simulink model "Standalone_CCSMPC_Controller"  (R2025b)
settings: Solver=FixedStepDiscrete  StartTime=0.0  StopTime=20  FixedStep=1e-4  MaxStep=1e-4  RelTol=1e-3
undefined symbols (not defined in the file): B_fric, J, Ld, Lq, PsiPM, Rs, Ts_ctrl, Ts_sim
libraries: simulink x1
settings Model: SimulationMode=processor-in-the-loop (pil)  Creator=Harish  LastModifiedBy=Harish
settings OptimizationCC: DefaultParameterBehavior=Inlined  EnhancedBackFolding=on  PassReuseOutputArgsAs=Individual arguments  ZeroExternalMemoryAtStartup=off  ZeroInternalMemoryAtStartup=off  OptimizeBlockOrder=speed  DifferentSizesBufferReuse=on  OptimizationCustomize=off  EfficientTunableParamExpr=on
settings DebuggingCC: ParameterTunabilityLossMsg=error
settings HardwareCC: TargetLargestAtomicInteger=Long  TargetLargestAtomicFloat=Double  TargetIntDivRoundTo=Zero  TargetEndianess=LittleEndian  TargetHWDeviceType=ARM Compatible->ARM Cortex-M
settings SFSimCC: MATLABDynamicMemAlloc=off
settings RTWCC: SystemTargetFile=ert.tlc  TemplateMakefile=ert_default_tmf  GenerateReport=on  Toolchain=MinGW64 | gmake (64-bit Windows)  GenerateCodeMetricsReport=on  Description=Embedded Coder
settings CodeAppCC: ForceParamTrailComments=on  IgnoreCustomStorageClasses=off  OperatorAnnotations=on  SimulinkDataObjDesc=on  SFDataObjDesc=on  InsertBlockDesc=on
settings ERTTargetCC: ERTCustomFileTemplate=example_file_process.tlc  TargetLangStandard=C99 (ISO)  GenerateSampleERTMain=on  SupportContinuousTime=on

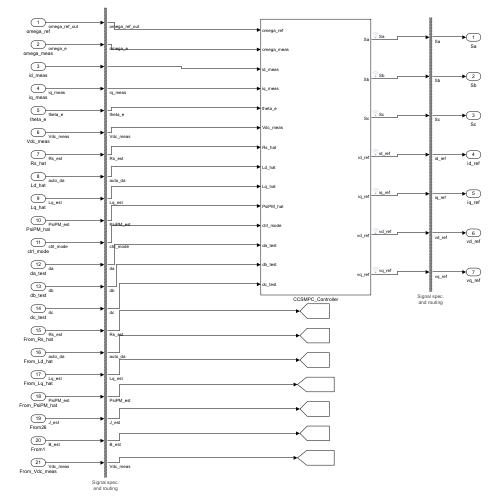
[thumbnail: Simulink's stored preview of the top-level diagram]
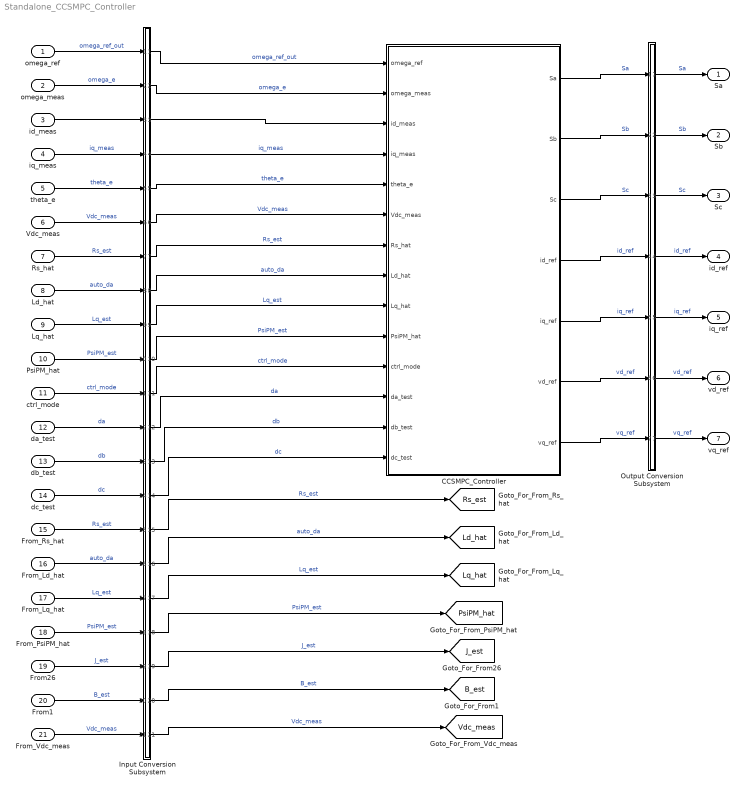
== system Standalone_CCSMPC_Controller ==
  omega_ref : Inport  OutDataTypeStr=double  PortDimensions=[1]  SampleTime=0.0001
  omega_meas : Inport  Port=2  OutDataTypeStr=double  PortDimensions=[1]  SampleTime=0.0001
  id_meas : Inport  Port=3  OutDataTypeStr=double  PortDimensions=[1]  SampleTime=0.0001
  iq_meas : Inport  Port=4  OutDataTypeStr=double  PortDimensions=[1]  SampleTime=0.0001
  theta_e : Inport  Port=5  OutDataTypeStr=double  PortDimensions=[1]  SampleTime=0.0001
  Vdc_meas : Inport  Port=6  OutDataTypeStr=double  PortDimensions=[1]  SampleTime=0.0001
  Rs_hat : Inport  Port=7  OutDataTypeStr=double  PortDimensions=[1]  SampleTime=0.0001
  Ld_hat : Inport  Port=8  OutDataTypeStr=double  PortDimensions=[1]  SampleTime=0.0001
  Lq_hat : Inport  Port=9  OutDataTypeStr=double  PortDimensions=[1]  SampleTime=0.0001
  PsiPM_hat : Inport  Port=10  OutDataTypeStr=double  PortDimensions=[1]  SampleTime=0.0001
  ctrl_mode : Inport  Port=11  OutDataTypeStr=double  PortDimensions=[1]  SampleTime=0.0001
  da_test : Inport  Port=12  OutDataTypeStr=double  PortDimensions=[1]  SampleTime=0.0001
  db_test : Inport  Port=13  OutDataTypeStr=double  PortDimensions=[1]  SampleTime=0.0001
  dc_test : Inport  Port=14  OutDataTypeStr=double  PortDimensions=[1]  SampleTime=0.0001
  From_Rs_hat : Inport  Port=15  OutDataTypeStr=double  PortDimensions=[1]  SampleTime=0.0001
  From_Ld_hat : Inport  Port=16  OutDataTypeStr=double  PortDimensions=[1]  SampleTime=0.0001
  From_Lq_hat : Inport  Port=17  OutDataTypeStr=double  PortDimensions=[1]  SampleTime=0.0001
  From_PsiPM_hat : Inport  Port=18  OutDataTypeStr=double  PortDimensions=[1]  SampleTime=0.0001
  From26 : Inport  Port=19  OutDataTypeStr=double  PortDimensions=[1]  SampleTime=0.0001
  From1 : Inport  Port=20  OutDataTypeStr=double  PortDimensions=[1]  SampleTime=0.0001
  From_Vdc_meas : Inport  Port=21  OutDataTypeStr=double  PortDimensions=[1]  SampleTime=0.0001
  CCSMPC_Controller : Subsystem
  Input Conversion Subsystem : Subsystem  Tag=__SLT_ICS__  Description=|
      | Signal spec.
      | and routing
      settings: AttributesFormatString=%<Description>
  Output Conversion Subsystem : Subsystem  Tag=__SLT_OCS__  Description=|
      | Signal spec.
      | and routing
      settings: AttributesFormatString=%<Description>
  Sa : Outport
  Sb : Outport  Port=2
  Sc : Outport  Port=3
  id_ref : Outport  Port=4
  iq_ref : Outport  Port=5
  vd_ref : Outport  Port=6
  vq_ref : Outport  Port=7
  tag scope: B_est=global, J_est=global, Ld_hat=global, Lq_hat=global, PsiPM_hat=global, Rs_est=global, Vdc_meas=global
  wires:
  omega_ref/1 -> Input Conversion Subsystem/1(Inport_1)  "omega_ref_out"
  omega_meas/1 -> Input Conversion Subsystem/2(Inport_2)  "omega_e"
  id_meas/1 -> Input Conversion Subsystem/3(Inport_3)
  iq_meas/1 -> Input Conversion Subsystem/4(Inport_4)  "iq_meas"
  theta_e/1 -> Input Conversion Subsystem/5(Inport_5)  "theta_e"
  Vdc_meas/1 -> Input Conversion Subsystem/6(Inport_6)  "Vdc_meas"
  Rs_hat/1 -> Input Conversion Subsystem/7(Inport_7)  "Rs_est"
  Ld_hat/1 -> Input Conversion Subsystem/8(Inport_8)  "auto_da"
  Lq_hat/1 -> Input Conversion Subsystem/9(Inport_9)  "Lq_est"
  PsiPM_hat/1 -> Input Conversion Subsystem/10(Inport_10)  "PsiPM_est"
  ctrl_mode/1 -> Input Conversion Subsystem/11(Inport_11)  "ctrl_mode"
  da_test/1 -> Input Conversion Subsystem/12(Inport_12)  "da"
  db_test/1 -> Input Conversion Subsystem/13(Inport_13)  "db"
  dc_test/1 -> Input Conversion Subsystem/14(Inport_14)  "dc"
  From_Rs_hat/1 -> Input Conversion Subsystem/15(Inport_15)  "Rs_est"
  From_Ld_hat/1 -> Input Conversion Subsystem/16(Inport_16)  "auto_da"
  From_Lq_hat/1 -> Input Conversion Subsystem/17(Inport_17)  "Lq_est"
  From_PsiPM_hat/1 -> Input Conversion Subsystem/18(Inport_18)  "PsiPM_est"
  From26/1 -> Input Conversion Subsystem/19(Inport_19)  "J_est"
  From1/1 -> Input Conversion Subsystem/20(Inport_20)  "B_est"
  From_Vdc_meas/1 -> Input Conversion Subsystem/21(Inport_21)  "Vdc_meas"
  Output Conversion Subsystem/1(Outport_1) -> Sa/1  "Sa"
  Output Conversion Subsystem/2(Outport_2) -> Sb/1  "Sb"
  Output Conversion Subsystem/3(Outport_3) -> Sc/1  "Sc"
  Output Conversion Subsystem/4(Outport_4) -> id_ref/1  "id_ref"
  Output Conversion Subsystem/5(Outport_5) -> iq_ref/1  "iq_ref"
  Output Conversion Subsystem/6(Outport_6) -> vd_ref/1  "vd_ref"
  Output Conversion Subsystem/7(Outport_7) -> vq_ref/1  "vq_ref"
  Input Conversion Subsystem/1(Outport_1) -> CCSMPC_Controller/1(omega_ref)  "omega_ref_out"
  Input Conversion Subsystem/2(Outport_2) -> CCSMPC_Controller/2(omega_meas)  "omega_e"
  Input Conversion Subsystem/3(Outport_3) -> CCSMPC_Controller/3(id_meas)
  Input Conversion Subsystem/4(Outport_4) -> CCSMPC_Controller/4(iq_meas)  "iq_meas"
  Input Conversion Subsystem/5(Outport_5) -> CCSMPC_Controller/5(theta_e)  "theta_e"
  Input Conversion Subsystem/6(Outport_6) -> CCSMPC_Controller/6(Vdc_meas)  "Vdc_meas"
  Input Conversion Subsystem/7(Outport_7) -> CCSMPC_Controller/7(Rs_hat)  "Rs_est"
  Input Conversion Subsystem/8(Outport_8) -> CCSMPC_Controller/8(Ld_hat)  "auto_da"
  Input Conversion Subsystem/9(Outport_9) -> CCSMPC_Controller/9(Lq_hat)  "Lq_est"
  Input Conversion Subsystem/10(Outport_10) -> CCSMPC_Controller/10(PsiPM_hat)  "PsiPM_est"
  Input Conversion Subsystem/11(Outport_11) -> CCSMPC_Controller/11(ctrl_mode)  "ctrl_mode"
  Input Conversion Subsystem/12(Outport_12) -> CCSMPC_Controller/12(da_test)  "da"
  Input Conversion Subsystem/13(Outport_13) -> CCSMPC_Controller/13(db_test)  "db"
  Input Conversion Subsystem/14(Outport_14) -> CCSMPC_Controller/14(dc_test)  "dc"
  Input Conversion Subsystem/15(Outport_15) -> [Rs_est]  "Rs_est"
  Input Conversion Subsystem/16(Outport_16) -> [Ld_hat]  "auto_da"
  Input Conversion Subsystem/17(Outport_17) -> [Lq_hat]  "Lq_est"
  Input Conversion Subsystem/18(Outport_18) -> [PsiPM_hat]  "PsiPM_est"
  Input Conversion Subsystem/19(Outport_19) -> [J_est]  "J_est"
  Input Conversion Subsystem/20(Outport_20) -> [B_est]  "B_est"
  Input Conversion Subsystem/21(Outport_21) -> [Vdc_meas]  "Vdc_meas"
  CCSMPC_Controller/1(Sa) -> Output Conversion Subsystem/1(Inport_1)  "Sa"
  CCSMPC_Controller/2(Sb) -> Output Conversion Subsystem/2(Inport_2)  "Sb"
  CCSMPC_Controller/3(Sc) -> Output Conversion Subsystem/3(Inport_3)  "Sc"
  CCSMPC_Controller/4(id_ref) -> Output Conversion Subsystem/4(Inport_4)  "id_ref"
  CCSMPC_Controller/5(iq_ref) -> Output Conversion Subsystem/5(Inport_5)  "iq_ref"
  CCSMPC_Controller/6(vd_ref) -> Output Conversion Subsystem/6(Inport_6)  "vd_ref"
  CCSMPC_Controller/7(vq_ref) -> Output Conversion Subsystem/7(Inport_7)  "vq_ref"

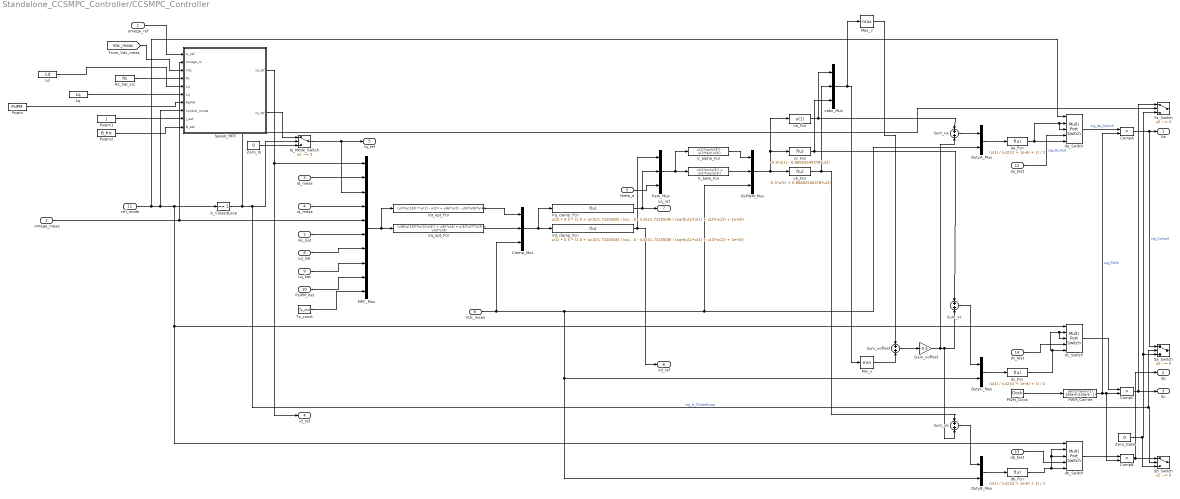
== system Standalone_CCSMPC_Controller/CCSMPC_Controller ==
  omega_ref : Inport  SampleTime=Ts_ctrl
  omega_meas : Inport  Port=2  SampleTime=Ts_ctrl
  id_meas : Inport  Port=3  SampleTime=Ts_ctrl
  iq_meas : Inport  Port=4  SampleTime=Ts_ctrl
  theta_e : Inport  Port=5  SampleTime=Ts_ctrl
  Vdc_meas : Inport  Port=6  SampleTime=Ts_ctrl
  Rs_hat : Inport  Port=7  SampleTime=Ts_ctrl
  Ld_hat : Inport  Port=8  SampleTime=Ts_ctrl
  Lq_hat : Inport  Port=9  SampleTime=Ts_ctrl
  PsiPM_hat : Inport  Port=10  SampleTime=Ts_ctrl
  ctrl_mode : Inport  Port=11  SampleTime=Ts_ctrl
  da_test : Inport  Port=12
  db_test : Inport  Port=13
  dc_test : Inport  Port=14
  Clamp_Mux : Mux  Inputs=3
  CompA : RelationalOperator  Operator=>  OutDataTypeStr=boolean  SampleTime=Ts_sim  RndMeth=Simplest  InputSameDT=off
  CompB : RelationalOperator  Operator=>  OutDataTypeStr=boolean  SampleTime=Ts_sim  RndMeth=Simplest  InputSameDT=off
  CompC : RelationalOperator  Operator=>  OutDataTypeStr=boolean  SampleTime=Ts_sim  RndMeth=Simplest  InputSameDT=off
  DutyA_Mux : Mux  Inputs=2
  DutyB_Mux : Mux  Inputs=2
  DutyC_Mux : Mux  Inputs=2
  Gain_voffset : Gain  Gain=-0.5
  Iq_Mode_Switch : Switch  Criteria=u2 ~= 0  Threshold=0.5  SaturateOnIntegerOverflow=off  InputSameDT=off
  Is_ClosedLoop : simulink/Logic and Bit Operations/Compare To Constant  relop===  const=1  OutDataTypeStr=boolean
  Ld : Constant  Value=Ld
  Lq : Constant  Value=Lq
  MPC_Mux : Mux  Inputs=10
  Max_v : MinMax  Function=max
  Min_v : MinMax
  PWM_Carrier : Fcn  Expr=abs(2*rem(u(1), 100e-6)/100e-6 - 1)
  PWM_Clock : DigitalClock  SampleTime=Ts_sim
  Park_Mux : Mux  Inputs=3
  Psipm : Constant  Value=PsiPM
  Psipm1 : Constant  Value=J
  Psipm2 : Constant  Value=B_fric
  Rs_hat_src : Constant  Value=Rs
  SVPWM_Mux : Mux  Inputs=3
  Sa_Switch : Switch  Criteria=u2 ~= 0  Threshold=0.5  SaturateOnIntegerOverflow=off  InputSameDT=off
  Sb_Switch : Switch  Criteria=u2 ~= 0  Threshold=0.5  SaturateOnIntegerOverflow=off  InputSameDT=off
  Sc_Switch : Switch  Criteria=u2 ~= 0  Threshold=0.5  SaturateOnIntegerOverflow=off  InputSameDT=off
  Speed_MPC : MATLAB Function  TreatAsAtomicUnit=on
  Sum_va : Sum
  Sum_vb : Sum
  Sum_vc : Sum
  Sum_voffset : Sum
  Ts_const : Constant  Value=Ts_ctrl  SampleTime=Ts_ctrl
  V_alpha_Fcn : Fcn  Expr=u(1)*cos(u(3)) - u(2)*sin(u(3))
  V_beta_Fcn : Fcn  Expr=u(1)*sin(u(3)) + u(2)*cos(u(3))
  Vd_clamp_Fcn : Fcn  Expr=u(1) * 0.5 * (1.0 + (u(3)/1.7320508) / (sqrt(u(1)*u(1) + u(2)*u(2)) + 1e-6) - abs(1.0 - (u(3)/1.7320508) / (sqrt(u(1)*u(1) + u(2)*u(2)) + 1e-6)))
  Vd_opt_Fcn : Fcn  Expr=(u(7)/u(10)) * (u(1) - u(2)) + u(6)*u(2) - u(5)*u(8)*u(4);
  Vq_clamp_Fcn : Fcn  Expr=u(2) * 0.5 * (1.0 + (u(3)/1.7320508) / (sqrt(u(1)*u(1) + u(2)*u(2)) + 1e-6) - abs(1.0 - (u(3)/1.7320508) / (sqrt(u(1)*u(1) + u(2)*u(2)) + 1e-6)))
  Vq_opt_Fcn : Fcn  Expr=(u(8)/u(10))*(u(3)-u(4)) + u(6)*u(4) + u(5)*u(7)*u(2) + u(5)*u(9)
  Zero_Gate : Constant  Value=0  OutDataTypeStr=boolean  SampleTime=Ts_ctrl
  Zero_Iq : Constant  Value=0  SampleTime=Ts_ctrl
  da_Fcn : Fcn  Expr=(u(1) / (u(2)/2 + 1e-6) + 1) / 2
  da_Switch : MultiPortSwitch  DataPortOrder=Zero-based contiguous  Inputs=4  DataPortIndices={1,4,2}  zeroidx=on  SaturateOnIntegerOverflow=off  InputSameDT=off
  db_Fcn : Fcn  Expr=(u(1) / (u(2)/2 + 1e-6) + 1) / 2
  db_Switch : MultiPortSwitch  DataPortOrder=Zero-based contiguous  Inputs=4  DataPortIndices={1,4,2}  zeroidx=on  SaturateOnIntegerOverflow=off  InputSameDT=off
  dc_Fcn : Fcn  Expr=(u(1) / (u(2)/2 + 1e-6) + 1) / 2
  dc_Switch : MultiPortSwitch  DataPortOrder=Zero-based contiguous  Inputs=4  DataPortIndices={1,4,2}  zeroidx=on  SaturateOnIntegerOverflow=off  InputSameDT=off
  va_Fcn : Fcn  Expr=u(1)
  vabc_Mux : Mux  Inputs=3
  vb_Fcn : Fcn  Expr=-0.5*u(1) + 0.86602540378*u(2)
  vc_Fcn : Fcn  Expr=-0.5*u(1) - 0.86602540378*u(2)
  Sa : Outport  SampleTime=Ts_ctrl
  Sb : Outport  Port=2  SampleTime=Ts_ctrl
  Sc : Outport  Port=3  SampleTime=Ts_ctrl
  id_ref : Outport  Port=4  SampleTime=Ts_ctrl
  iq_ref : Outport  Port=5  SampleTime=Ts_ctrl
  vd_ref : Outport  Port=6  SampleTime=Ts_ctrl
  vq_ref : Outport  Port=7  SampleTime=Ts_ctrl
  wires:
  Min_v/1 -> Sum_voffset/2
  SVPWM_Mux/1 -> va_Fcn/1, vc_Fcn/1, vb_Fcn/1
  omega_meas/1 -> Speed_MPC/2(omega_m), MPC_Mux/5
  Ld/1 -> Speed_MPC/5(Ld)
  db_Switch/1 -> CompB/1
  [Vdc_meas] -> Speed_MPC/3(Vdc)
  Park_Mux/1 -> V_alpha_Fcn/1, V_beta_Fcn/1
  Iq_Mode_Switch/1 -> MPC_Mux/3, iq_ref/1
  Rs_hat_src/1 -> Speed_MPC/4(Rs)
  Sum_va/1 -> DutyA_Mux/1
  Vq_opt_Fcn/1 -> Clamp_Mux/2
  Lq/1 -> Speed_MPC/6(Lq)
  Zero_Gate/1 -> Sa_Switch/3, Sc_Switch/3, Sb_Switch/3
  V_beta_Fcn/1 -> SVPWM_Mux/2
  Psipm/1 -> Speed_MPC/7(PsiPM)
  Vd_opt_Fcn/1 -> Clamp_Mux/1
  ctrl_mode/1 -> dc_Switch/1, db_Switch/1, Is_ClosedLoop/1, Speed_MPC/8(control_mode), da_Switch/1
  Speed_MPC/1(id_ref) -> MPC_Mux/1, id_ref/1
  Vd_clamp_Fcn/1 -> vd_ref/1, Park_Mux/1
  Speed_MPC/2(iq_ref) -> Iq_Mode_Switch/1
  Zero_Iq/1 -> Iq_Mode_Switch/3
  id_meas/1 -> MPC_Mux/2
  Is_ClosedLoop/1 -> Sb_Switch/2, Sa_Switch/2, Iq_Mode_Switch/2, Sc_Switch/2  "sig_Is_ClosedLoop"
  iq_meas/1 -> MPC_Mux/4
  Gain_voffset/1 -> Sum_vb/2, Sum_vc/2, Sum_va/2
  Rs_hat/1 -> MPC_Mux/6
  da_test/1 -> da_Switch/4  "sig_da_test"
  Ld_hat/1 -> MPC_Mux/7
  db_test/1 -> db_Switch/4
  Clamp_Mux/1 -> Vd_clamp_Fcn/1, Vq_clamp_Fcn/1
  Lq_hat/1 -> MPC_Mux/8
  PsiPM_hat/1 -> MPC_Mux/9
  dc_test/1 -> dc_Switch/4
  Ts_const/1 -> MPC_Mux/10
  MPC_Mux/1 -> Vq_opt_Fcn/1, Vd_opt_Fcn/1
  Vdc_meas/1 -> DutyC_Mux/2, DutyB_Mux/2, DutyA_Mux/2, SVPWM_Mux/3, Clamp_Mux/3
  theta_e/1 -> Park_Mux/3
  dc_Fcn/1 -> dc_Switch/5, dc_Switch/3, dc_Switch/2
  Vq_clamp_Fcn/1 -> Park_Mux/2, vq_ref/1
  V_alpha_Fcn/1 -> SVPWM_Mux/1
  da_Switch/1 -> CompA/1  "sig_da_Switch"
  va_Fcn/1 -> Sum_va/1, vabc_Mux/1
  vc_Fcn/1 -> Sum_vc/1, vabc_Mux/3
  vb_Fcn/1 -> Sum_vb/1, vabc_Mux/2
  vabc_Mux/1 -> Min_v/1, Max_v/1
  Max_v/1 -> Sum_voffset/1
  Sum_voffset/1 -> Gain_voffset/1
  Sum_vc/1 -> DutyC_Mux/1
  DutyC_Mux/1 -> dc_Fcn/1
  Sum_vb/1 -> DutyB_Mux/1
  DutyA_Mux/1 -> da_Fcn/1
  CompA/1 -> Sa/1, Sa_Switch/1  "sig_CompA"
  DutyB_Mux/1 -> db_Fcn/1
  da_Fcn/1 -> da_Switch/5, da_Switch/3, da_Switch/2
  PWM_Clock/1 -> PWM_Carrier/1
  CompC/1 -> Sc_Switch/1, Sc/1
  db_Fcn/1 -> db_Switch/5, db_Switch/2, db_Switch/3
  dc_Switch/1 -> CompC/1
  PWM_Carrier/1 -> CompB/2, CompC/2, CompA/2  "sig_PWM"
  CompB/1 -> Sb/1, Sb_Switch/1
  omega_ref/1 -> Speed_MPC/1(w_ref)
  Psipm1/1 -> Speed_MPC/9(J_est)
  Psipm2/1 -> Speed_MPC/10(B_est)

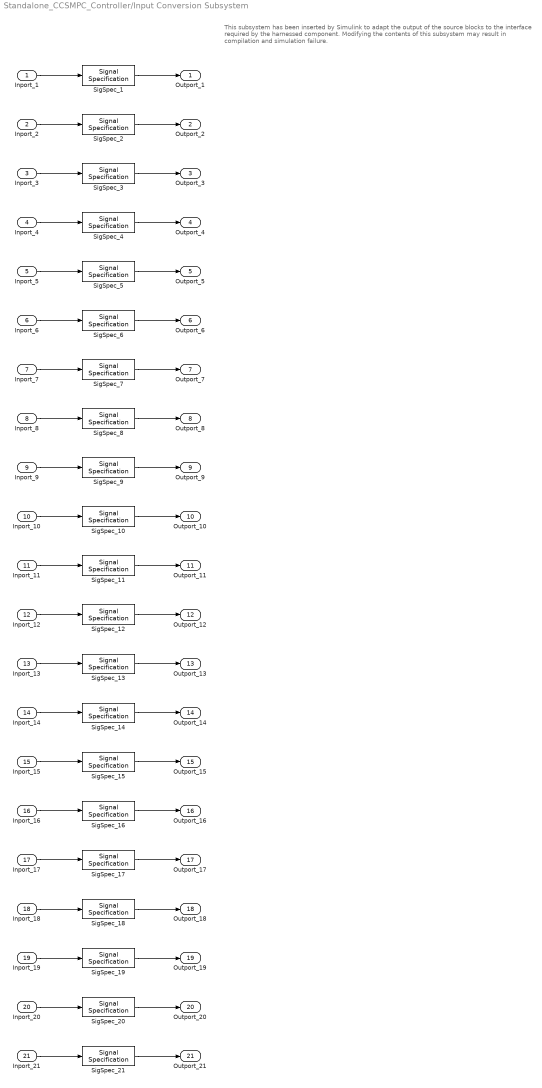
== system Standalone_CCSMPC_Controller/Input Conversion Subsystem ==
  note: This subsystem has been inserted by Simulink to adapt the output of the source blocks to the interface required by the harnessed component.
      |  Modifying the contents of this subsystem may result in compilation and simulation failure.
  Inport_1 : Inport
  Inport_2 : Inport  Port=2
  Inport_3 : Inport  Port=3
  Inport_4 : Inport  Port=4
  Inport_5 : Inport  Port=5
  Inport_6 : Inport  Port=6
  Inport_7 : Inport  Port=7
  Inport_8 : Inport  Port=8
  Inport_9 : Inport  Port=9
  Inport_10 : Inport  Port=10
  Inport_11 : Inport  Port=11
  Inport_12 : Inport  Port=12
  Inport_13 : Inport  Port=13
  Inport_14 : Inport  Port=14
  Inport_15 : Inport  Port=15
  Inport_16 : Inport  Port=16
  Inport_17 : Inport  Port=17
  Inport_18 : Inport  Port=18
  Inport_19 : Inport  Port=19
  Inport_20 : Inport  Port=20
  Inport_21 : Inport  Port=21
  SigSpec_{1..21} (21 alike) : SignalSpecification  OutDataTypeStr=double  Dimensions=[1]
  Outport_1 : Outport
  Outport_2 : Outport  Port=2
  Outport_3 : Outport  Port=3
  Outport_4 : Outport  Port=4
  Outport_5 : Outport  Port=5
  Outport_6 : Outport  Port=6
  Outport_7 : Outport  Port=7
  Outport_8 : Outport  Port=8
  Outport_9 : Outport  Port=9
  Outport_10 : Outport  Port=10
  Outport_11 : Outport  Port=11
  Outport_12 : Outport  Port=12
  Outport_13 : Outport  Port=13
  Outport_14 : Outport  Port=14
  Outport_15 : Outport  Port=15
  Outport_16 : Outport  Port=16
  Outport_17 : Outport  Port=17
  Outport_18 : Outport  Port=18
  Outport_19 : Outport  Port=19
  Outport_20 : Outport  Port=20
  Outport_21 : Outport  Port=21
  wires:
  SigSpec_1/1 -> Outport_1/1
  Inport_1/1 -> SigSpec_1/1
  SigSpec_2/1 -> Outport_2/1
  Inport_2/1 -> SigSpec_2/1
  SigSpec_3/1 -> Outport_3/1
  Inport_3/1 -> SigSpec_3/1
  SigSpec_4/1 -> Outport_4/1
  Inport_4/1 -> SigSpec_4/1
  SigSpec_5/1 -> Outport_5/1
  Inport_5/1 -> SigSpec_5/1
  SigSpec_6/1 -> Outport_6/1
  Inport_6/1 -> SigSpec_6/1
  SigSpec_7/1 -> Outport_7/1
  Inport_7/1 -> SigSpec_7/1
  SigSpec_8/1 -> Outport_8/1
  Inport_8/1 -> SigSpec_8/1
  SigSpec_9/1 -> Outport_9/1
  Inport_9/1 -> SigSpec_9/1
  SigSpec_10/1 -> Outport_10/1
  Inport_10/1 -> SigSpec_10/1
  SigSpec_11/1 -> Outport_11/1
  Inport_11/1 -> SigSpec_11/1
  SigSpec_12/1 -> Outport_12/1
  Inport_12/1 -> SigSpec_12/1
  SigSpec_13/1 -> Outport_13/1
  Inport_13/1 -> SigSpec_13/1
  SigSpec_14/1 -> Outport_14/1
  Inport_14/1 -> SigSpec_14/1
  SigSpec_15/1 -> Outport_15/1
  Inport_15/1 -> SigSpec_15/1
  SigSpec_16/1 -> Outport_16/1
  Inport_16/1 -> SigSpec_16/1
  SigSpec_17/1 -> Outport_17/1
  Inport_17/1 -> SigSpec_17/1
  SigSpec_18/1 -> Outport_18/1
  Inport_18/1 -> SigSpec_18/1
  SigSpec_19/1 -> Outport_19/1
  Inport_19/1 -> SigSpec_19/1
  SigSpec_20/1 -> Outport_20/1
  Inport_20/1 -> SigSpec_20/1
  SigSpec_21/1 -> Outport_21/1
  Inport_21/1 -> SigSpec_21/1

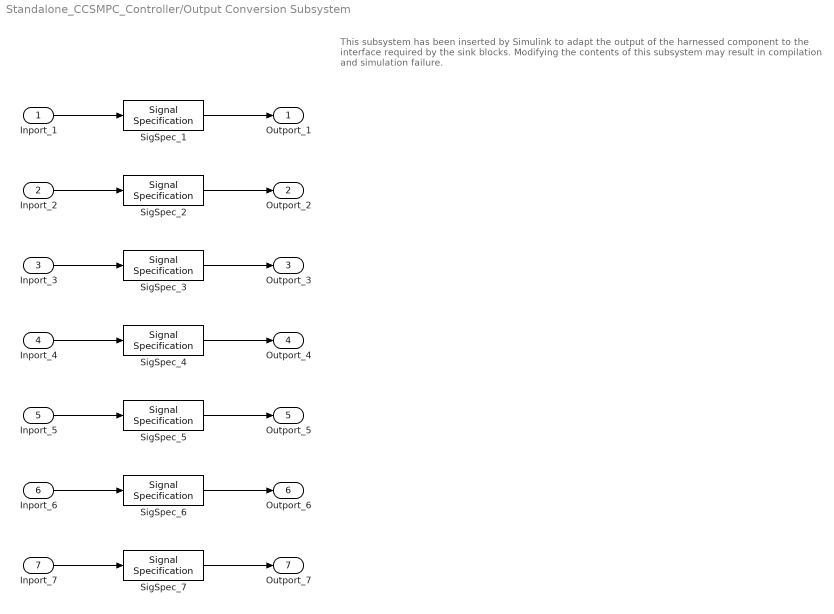
== system Standalone_CCSMPC_Controller/Output Conversion Subsystem ==
  note: This subsystem has been inserted by Simulink to adapt the output of the harnessed component to the interface required by the sink blocks.
      |  Modifying the contents of this subsystem may result in compilation and simulation failure.
  Inport_1 : Inport
  Inport_2 : Inport  Port=2
  Inport_3 : Inport  Port=3
  Inport_4 : Inport  Port=4
  Inport_5 : Inport  Port=5
  Inport_6 : Inport  Port=6
  Inport_7 : Inport  Port=7
  SigSpec_1 : SignalSpecification  OutDataTypeStr=boolean  Dimensions=[1]
  SigSpec_2 : SignalSpecification  OutDataTypeStr=boolean  Dimensions=[1]
  SigSpec_3 : SignalSpecification  OutDataTypeStr=boolean  Dimensions=[1]
  SigSpec_{4..7} (4 alike) : SignalSpecification  OutDataTypeStr=double  Dimensions=[1]
  Outport_1 : Outport
  Outport_2 : Outport  Port=2
  Outport_3 : Outport  Port=3
  Outport_4 : Outport  Port=4
  Outport_5 : Outport  Port=5
  Outport_6 : Outport  Port=6
  Outport_7 : Outport  Port=7
  wires:
  Inport_1/1 -> SigSpec_1/1
  SigSpec_1/1 -> Outport_1/1
  Inport_2/1 -> SigSpec_2/1
  SigSpec_2/1 -> Outport_2/1
  Inport_3/1 -> SigSpec_3/1
  SigSpec_3/1 -> Outport_3/1
  Inport_4/1 -> SigSpec_4/1
  SigSpec_4/1 -> Outport_4/1
  Inport_5/1 -> SigSpec_5/1
  SigSpec_5/1 -> Outport_5/1
  Inport_6/1 -> SigSpec_6/1
  SigSpec_6/1 -> Outport_6/1
  Inport_7/1 -> SigSpec_7/1
  SigSpec_7/1 -> Outport_7/1

== matlab function Standalone_CCSMPC_Controller/CCSMPC_Controller/Speed_MPC ==
  data: w_ref input double size=1; id_ref output double size=1; omega_m input double size=1; Vdc input double size=1; Rs input double size=1; Ld input double size=1; Lq input double size=1; PsiPM input double size=1; iq_ref output double size=1; control_mode input; J_est input; B_est input
function [id_ref, iq_ref] = Outer_MPC(w_ref, omega_m, Vdc, Rs, Ld, Lq, PsiPM, control_mode, J_est, B_est)
    % Cascaded Multi-Rate Speed MPC & MTPA/FW Joint Optimizer
    % control_mode: 1 = Active Speed Control, 0 = Disabled (Outputs 0 currents)
    
    id_ref = zeros(1, 1, 'double');
    iq_ref = zeros(1, 1, 'double');
    
    Ts_outer = 1e-3; % 1 kHz outer loop
    pp = 6; % i3 motor pole pairs
    I_max = 565.0; % Maximum inverter phase current (A peak)
    
    % --- Convert Electrical Speeds to Mechanical for MPC Model ---
    omega_mech = double(omega_m) / pp;
    w_ref_mech = double(w_ref) / pp;
    
    persistent omega_prev;
    persistent Te_prev;
    
    if isempty(omega_prev)
        omega_prev = omega_mech;
        Te_prev = 0.0;
    end
    
    % --- Control Mode Bypass ---
    if control_mode ~= 1
        omega_prev = omega_mech;
        Te_prev = 0.0;
        id_ref(1) = 0.0;
        iq_ref(1) = 0.0;
        return;
    end
    
    % --- Safety Clamps for Auto-Tuned Parameters ---
    J_val = max(double(J_est), 0.0001);
    B_val = max(double(B_est), 0.0);
    Psi_val = max(double(PsiPM), 0.01);
    Ld_val = max(double(Ld), 1e-6);
    Lq_val = max(double(Lq), 1e-6);
    
    % --- Outer Speed MPC (Incremental Model) ---
    d_omega = omega_mech - omega_prev;
    e_w = w_ref_mech - omega_mech;
    
    Am = 1.0 - (B_val * Ts_outer) / J_val;
    Bm = Ts_outer / J_val;
    
    % Tuned Cost function weights: fast disturbance rejection without sluggish lag
    Q_mpc = 1.0;
    R_mpc = 0.0001;
    
    % Error prediction
    E = e_w - Am * d_omega;
    
    % Optimal control move
    delta_Te = (Q_mpc * Bm) / (Q_mpc * Bm^2 + R_mpc) * E;
    Te_ref = Te_prev + delta_Te;
    
    % Dynamic Torque limits (allow up to 280 Nm peak acceleration torque)
    if Te_ref > 280.0, Te_ref = 280.0; end
    if Te_ref < -280.0, Te_ref = -280.0; end
    
    % Update state for next step
    omega_prev = omega_mech;
    Te_prev = Te_ref;
    
    % --- Exact MTPA Current Allocation (Analytic Current Vector Optimization) ---
    dL = Lq_val - Ld_val;
    
    if abs(Te_ref) < 1e-3 || dL < 1e-7
        id_mtpa = 0.0;
        iq_mtpa = Te_ref / (1.5 * pp * Psi_val);
    else
        % Solve for current magnitude Is along MTPA trajectory
        Is_est = min(I_max, max(0.0, abs(Te_ref) / (1.5 * pp * Psi_val)));
        
        for iter = 1:8
            if Is_est < 1e-2, Is_est = 1e-2; end
            term_sq = sqrt(Psi_val^2 + 8.0 * (dL^2) * (Is_est^2));
            sin_g = (-Psi_val + term_sq) / (4.0 * dL * Is_est);
            if sin_g < 0.0, sin_g = 0.0; end
            if sin_g > 1.0, sin_g = 1.0; end
            cos_g = sqrt(max(0.0, 1.0 - sin_g^2));
            
            id_k = -Is_est * sin_g;
            iq_k = Is_est * cos_g;
            
            Te_k = 1.5 * pp * (Psi_val * iq_k + (Ld_val - Lq_val) * id_k * iq_k);
            err_t = Te_k - abs(Te_ref);
            if abs(err_t) < 0.05, break; end
            
            dTe_dIs = 1.5 * pp * (Psi_val * cos_g + 2.0 * dL * Is_est * sin_g * cos_g);
            if abs(dTe_dIs) < 1e-3, break; end
            
            Is_est = max(0.0, min(I_max, Is_est - err_t / dTe_dIs));
        end
        
        term_sq = sqrt(Psi_val^2 + 8.0 * (dL^2) * (Is_est^2));
        sin_g = (-Psi_val + term_sq) / (4.0 * dL * Is_est);
        if sin_g < 0.0, sin_g = 0.0; end
        if sin_g > 1.0, sin_g = 1.0; end
        cos_g = sqrt(max(0.0, 1.0 - sin_g^2));
        
        id_mtpa = -Is_est * sin_g;
        if Te_ref >= 0.0
            iq_mtpa = Is_est * cos_g;
        else
            iq_mtpa = -Is_est * cos_g;
        end
    end
    
    % --- High Speed Field Weakening (Only Active When Rotor Spun Up) ---
    V_max = (double(Vdc) / sqrt(3.0)) * 0.95;
    omega_e = max(abs(double(omega_m)), 1.0);
    
    Vd_est = -omega_e * Lq_val * iq_mtpa;
    Vq_est = omega_e * Ld_val * id_mtpa + omega_e * Psi_val;
    V_est = sqrt(Vd_est^2 + Vq_est^2);
    
    if V_est > V_max && double(omega_m) > 150.0
        % FW Demagnetization Search
        id_fw = id_mtpa;
        V_limit2 = (V_max / omega_e)^2;
        K_t = 1.5 * pp;
        
        for iter = 1:8
            denom = Psi_val + (Ld_val - Lq_val) * id_fw;
            if abs(denom) < 1e-4, denom = 1e-4; end
            iq_fw = Te_ref / (K_t * denom);
            
            f_val = (Ld_val * id_fw + Psi_val)^2 + (Lq_val * iq_fw)^2 - V_limit2;
            diq_did = -iq_fw * (Ld_val - Lq_val) / denom;
            df_did = 2.0 * Ld_val * (Ld_val * id_fw + Psi_val) + 2.0 * (Lq_val^2) * iq_fw * diq_did;
            if abs(df_did) < 1e-6, break; end
            
            id_fw_new = id_fw - f_val / df_did;
            if id_fw_new < -Psi_val / Ld_val, id_fw_new = -Psi_val / Ld_val; end
            if abs(id_fw_new - id_fw) < 1e-3
                id_fw = id_fw_new;
                break;
            end
            id_fw = id_fw_new;
        end
        id_out = id_fw;
        iq_out = Te_ref / (K_t * (Psi_val + (Ld_val - Lq_val) * id_out));
    else
        id_out = id_mtpa;
        iq_out = iq_mtpa;
    end
    
    % Final Safety Circle Clamp
    I_tot = sqrt(id_out^2 + iq_out^2);
    if I_tot > I_max
        scale = I_max / I_tot;
        id_out = id_out * scale;
        iq_out = iq_out * scale;
    end
    
    id_ref(1) = id_out;
    iq_ref(1) = iq_out;
end
